simulink model "Priority_demo"  (R2021a)
settings: Solver=FixedStepDiscrete  StartTime=0.0  StopTime=10.0  RelTol=1e-3
CloseFcn:
  | clear all
  | try
  | rmdir slprj\ s
  | catch
  | end
  | try
  | folder_name = [bdroot '*'];
  | rmdir(folder_name,'s')
  | catch
  | end
  | try
  | file_temp_name = [bdroot '.slxc'];
  | delete(file_temp_name)
  | %%delete *.mexw64
  | catch
  | end
  | clear folder_name file_temp_name
settings Model: Creator=jetson  LastModifiedBy=jetson
settings DataIOCC: SaveOutput=off  SignalLogging=off  DSMLogging=off  SaveTime=off  ReturnWorkspaceOutputs=off
settings OptimizationCC: DefaultParameterBehavior=Inlined  EnhancedBackFolding=on  PassReuseOutputArgsAs=Individual arguments  ZeroExternalMemoryAtStartup=off  ZeroInternalMemoryAtStartup=off  OptimizeBlockOrder=speed  DifferentSizesBufferReuse=on  OptimizationCustomize=off  EfficientTunableParamExpr=on
settings DebuggingCC: ParameterTunabilityLossMsg=error
settings SFSimCC: MATLABDynamicMemAlloc=off
settings RTWCC: SystemTargetFile=ert.tlc  GenCodeOnly=on  TemplateMakefile=ert_default_tmf  GenerateReport=on  RetainRTWFile=on  RTWUseSimCustomCode=on  IncludeHyperlinkInReport=on  LaunchReport=on  GenerateTraceInfo=on
settings CodeAppCC: ForceParamTrailComments=on  IgnoreCustomStorageClasses=off  OperatorAnnotations=on  SimulinkDataObjDesc=on  SFDataObjDesc=on  InsertBlockDesc=on
settings ERTTargetCC: TargetLangStandard=C99 (ISO)  GenerateSampleERTMain=on  InlinedParameterPlacement=NonHierarchical  ERTCustomFileTemplate=example_file_process.tlc

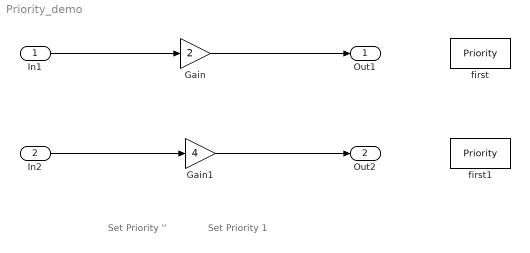
== system Priority_demo ==
  note: Set Priority 1
  note: Set Priority ''
  In1 : Inport
      settings: AttributesFormatString=Priority = %<Priority>
  In2 : Inport  Priority=1  Port=2
      settings: AttributesFormatString=Priority = %<Priority>
  Gain : Gain  Gain=2
      settings: AttributesFormatString=Priority = %<Priority>
  Gain1 : Gain  Priority=1  Gain=4
      settings: AttributesFormatString=Priority = %<Priority>
  first : S-Function  Priority=2  FunctionName=Priority  Parameters=pri  SFunctionDeploymentMode=off  EnableBusSupport=off  mask{pri=2}
      mask prompts: pri "prioriry"
      settings: AttributesFormatString=Priority = %<Priority>
      mask Callback pri: set(gcbh,'Priority', get(gcbh, 'pri'))
  first1 : S-Function  Priority=5  FunctionName=Priority  Parameters=pri  SFunctionDeploymentMode=off  EnableBusSupport=off  mask{pri=5}
      mask prompts: pri "prioriry"
      settings: AttributesFormatString=Priority = %<Priority>
      mask Callback pri: set(gcbh,'Priority', get(gcbh, 'pri'))
  Out1 : Outport
      settings: AttributesFormatString=Priority = %<Priority>
  Out2 : Outport  Priority=1  Port=2
      settings: AttributesFormatString=Priority = %<Priority>
  wires:
  In1/1 -> Gain/1
  Gain/1 -> Out1/1
  In2/1 -> Gain1/1
  Gain1/1 -> Out2/1
